simulink model "cprograminsimulink"  (R2018b)
settings: Solver=VariableStepAuto  StartTime=0.0  StopTime=10.0  RelTol=1e-3
settings Model: Creator=student  LastModifiedBy=student

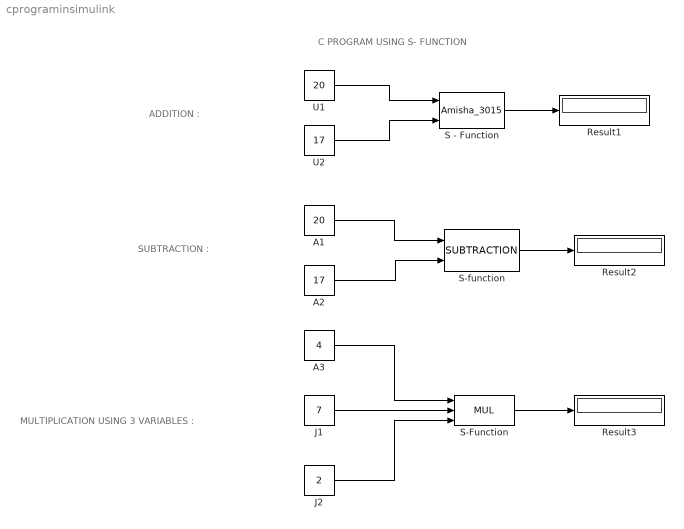
== system cprograminsimulink ==
  note: MULTIPLICATION USING 3 VARIABLES :
  note: SUBTRACTION :
  note: ADDITION :
  note: C PROGRAM USING S- FUNCTION
  A1 : Constant  Value=20
  A2 : Constant  Value=17
  A3 : Constant  Value=4
  J1 : Constant  Value=7
  J2 : Constant  Value=2
  Result1 : Display
  Result2 : Display
  Result3 : Display
  S - Function : S-Function  FunctionName=Amisha_3015  SFunctionDeploymentMode=off  EnableBusSupport=off
  S-Function : S-Function  FunctionName=MUL  SFunctionDeploymentMode=off  EnableBusSupport=off
  S-function : S-Function  FunctionName=SUBTRACTION  SFunctionDeploymentMode=off  EnableBusSupport=off
  U1 : Constant  Value=20
  U2 : Constant  Value=17
  wires:
  U1/1 -> S - Function/1
  U2/1 -> S - Function/2
  S - Function/1 -> Result1/1
  A1/1 -> S-function/1
  A2/1 -> S-function/2
  S-function/1 -> Result2/1
  S-Function/1 -> Result3/1
  A3/1 -> S-Function/1
  J1/1 -> S-Function/2
  J2/1 -> S-Function/3
